simulink subsystem "foc_hall_algorithm"  (R2021b)
settings: Solver=VariableStepAuto  StartTime=0.0  StopTime=10.0  RelTol=1e-3
values from neighbouring files (symbols this model uses):
  PI_params = mcb.internal.SetControllerParameters(pmsm,inverter,PU_System,T_pwm,2*Ts,Ts_speed)    [mcb_pmsm_foc_dual_f28379d_data.m]    (also in mcb_pmsm_foc_dual_f28379d_datascript.m; mcb_pmsm_foc_f280049C_data.m = mcb.internal.SetControllerParameters(pmsm,inverter,PU_System; mcb_pmsm_foc_f28335_data.m = mcb.internal.SetControllerParameters(pmsm,inverter,PU_System; mcb_pmsm_foc_hall_f28035_data.m = mcb.internal.SetControllerParameters(pmsm,inverter,PU_System)
  Ts = 5e-8    (= 5e-08)    [DCDC_Buck_Param.m]    (also in mcb_c2000_open_loop_control_data.m = T_pwm; mcb_c2000_pmsm_offset_data.m = T_pwm; mcb_pmsm_foc_dual_f28379d_data.m = 5e-05; mcb_pmsm_foc_dual_f28379d_datascript.m = 5e-05)
  Ts_speed = 20*Ts    (= 0.001)    [mcb_pmsm_foc_dual_f28379d_data.m]    (also in mcb_pmsm_foc_dual_f28379d_datascript.m; mcb_pmsm_foc_f280049C_data.m = 0.0005; mcb_pmsm_foc_f28335_data.m = 0.0005; mcb_pmsm_foc_hall_f28035_data.m = 0.0005)
libraries: demo_controls x1
settings Model: Creator=The MathWorks, Inc.  LastModifiedBy=The MathWorks, Inc.
settings SolverCC: AlgebraicLoopSolver=TrustRegion
settings DebuggingCC: SFMachineParentedDataDiag=warning

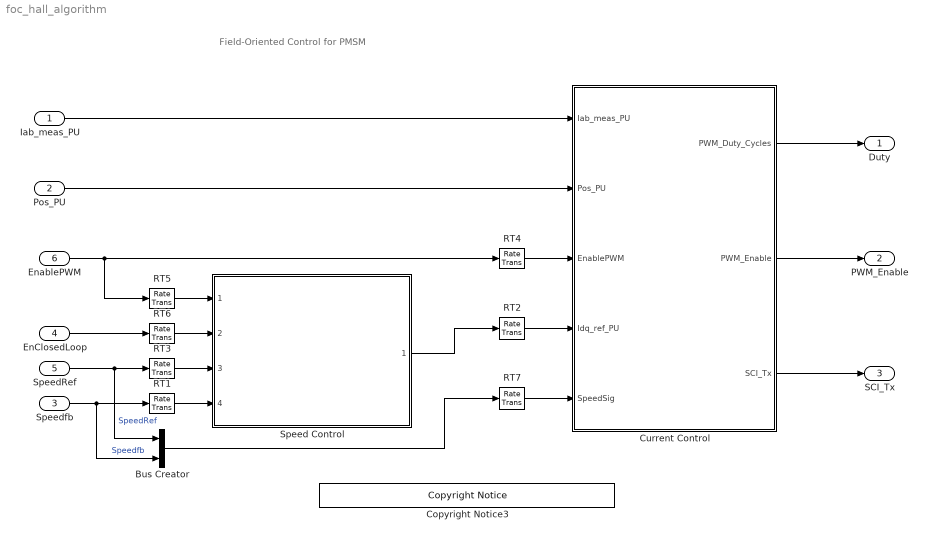
== system foc_hall_algorithm ==
  note: Field-Oriented Control for PMSM
  Iab_meas_PU : Inport
  Pos_PU : Inport  Port=2
  Speedfb : Inport  Port=3
  EnClosedLoop : Inport  Port=4
  SpeedRef : Inport  Port=5
  EnablePWM : Inport  Port=6
  Bus Creator : BusCreator  Inputs=2
  Copyright Notice3 : demo_controls/Copyright Notice  year=2020  prod=tic2000
      settings: SourceProductBaseCode=ME
  Current Control : Subsystem  TreatAsAtomicUnit=on
      settings: RTWSystemCode=Nonreusable function
  RT{1,3,5..6} (4 alike) : RateTransition  Deterministic=off  OutPortSampleTime=Ts_speed
  RT2 : RateTransition  Integrity=off  Deterministic=off  OutPortSampleTime=Ts
  RT4 : RateTransition  Deterministic=off
  RT7 : RateTransition  Integrity=off  Deterministic=off  OutPortSampleTime=Ts
  Speed Control : Subsystem  TreatAsAtomicUnit=on  SystemSampleTime=Ts_speed  ReferencedSubsystem=speed_control  Kp_speed=PI_params.Kp_speed  Ki_speed=PI_params.Ki_speed*Ts_speed
  Duty : Outport  InitialOutput=0  VectorParamsAs1DForOutWhenUnconnected=off
  PWM_Enable : Outport  Port=2  InitialOutput=0  VectorParamsAs1DForOutWhenUnconnected=off
  SCI_Tx : Outport  Port=3  InitialOutput=0  VectorParamsAs1DForOutWhenUnconnected=off
  wires:
  RT6/1 -> Speed Control/2
  Speed Control/1 -> RT2/1
  RT2/1 -> Current Control/4(Idq_ref_PU)
  Current Control/1(PWM_Duty_Cycles) -> Duty/1
  RT1/1 -> Speed Control/4
  RT5/1 -> Speed Control/1
  Current Control/2(PWM_Enable) -> PWM_Enable/1
  Pos_PU/1 -> Current Control/2(Pos_PU)
  RT3/1 -> Speed Control/3
  EnClosedLoop/1 -> RT6/1
  Iab_meas_PU/1 -> Current Control/1(Iab_meas_PU)
  EnablePWM/1 -> RT5/1, RT4/1
  RT4/1 -> Current Control/3(EnablePWM)
  Current Control/3(SCI_Tx) -> SCI_Tx/1
  Bus Creator/1 -> RT7/1
  Speedfb/1 -> Bus Creator/2, RT1/1  "Speedfb"
  SpeedRef/1 -> Bus Creator/1, RT3/1  "SpeedRef"
  RT7/1 -> Current Control/5(SpeedSig)

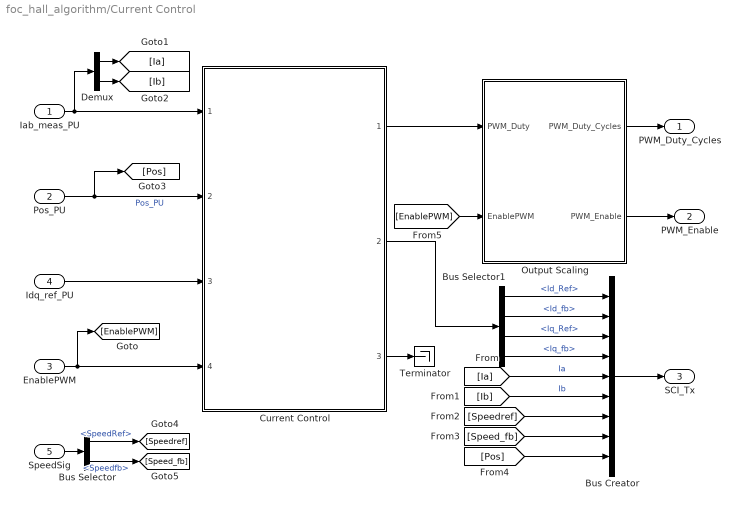
== system foc_hall_algorithm/Current Control ==
  Iab_meas_PU : Inport
  Pos_PU : Inport  Port=2
  EnablePWM : Inport  Port=3
  Idq_ref_PU : Inport  Port=4
  SpeedSig : Inport  Port=5
  Bus Creator : BusCreator  Inputs=9
  Bus Selector : BusSelector  OutputSignals=SpeedRef,Speedfb
  Bus Selector1 : BusSelector  OutputSignals=Id_Ref,Id_fb,Iq_Ref,Iq_fb
  Current Control : Subsystem  ReferencedSubsystem=current_control  Kpd=PI_params.Kp_i  Kid=PI_params.Ki_i*Ts  Kpq=PI_params.Kp_i  Kiq=PI_params.Ki_i*Ts
  Demux : Demux  Outputs=2
  Output Scaling : Subsystem
  Terminator : Terminator
  PWM_Duty_Cycles : Outport
  PWM_Enable : Outport  Port=2
  SCI_Tx : Outport  Port=3
  wires:
  Output Scaling/2(PWM_Enable) -> PWM_Enable/1
  Pos_PU/1 -> [Pos], Current Control/2  "Pos_PU"
  Output Scaling/1(PWM_Duty_Cycles) -> PWM_Duty_Cycles/1
  EnablePWM/1 -> Current Control/4, [EnablePWM]
  Idq_ref_PU/1 -> Current Control/3
  Current Control/1 -> Output Scaling/1(PWM_Duty)
  Iab_meas_PU/1 -> Current Control/1, Demux/1
  [Pos] -> Bus Creator/9
  [Ib] -> Bus Creator/6  "Ib"
  [Speed_fb] -> Bus Creator/8
  Current Control/2 -> Bus Selector1/1
  [Ia] -> Bus Creator/5  "Ia"
  Bus Selector1/4 -> Bus Creator/4  "<Iq_fb>"
  Bus Selector1/3 -> Bus Creator/3  "<Iq_Ref>"
  Bus Selector1/1 -> Bus Creator/1  "<Id_Ref>"
  [Speedref] -> Bus Creator/7
  Bus Selector1/2 -> Bus Creator/2  "<Id_fb>"
  Bus Creator/1 -> SCI_Tx/1
  [EnablePWM] -> Output Scaling/2(EnablePWM)
  Demux/1 -> [Ia]
  Demux/2 -> [Ib]
  SpeedSig/1 -> Bus Selector/1
  Bus Selector/1 -> [Speedref]  "<SpeedRef>"
  Bus Selector/2 -> [Speed_fb]  "<Speedfb>"
  Current Control/3 -> Terminator/1

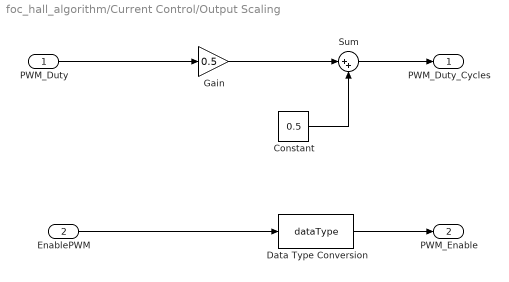
== system foc_hall_algorithm/Current Control/Output Scaling ==
  PWM_Duty : Inport
  EnablePWM : Inport  Port=2
  Constant : Constant  Value=0.5  OutDataTypeStr=dataType
  Data Type Conversion : DataTypeConversion  OutDataTypeStr=dataType
  Gain : Gain  Gain=0.5  OutDataTypeStr=Inherit: Same as input
  Sum : Sum  Inputs=|++
  PWM_Duty_Cycles : Outport
  PWM_Enable : Outport  Port=2
  wires:
  EnablePWM/1 -> Data Type Conversion/1
  Data Type Conversion/1 -> PWM_Enable/1
  PWM_Duty/1 -> Gain/1
  Gain/1 -> Sum/1
  Constant/1 -> Sum/2
  Sum/1 -> PWM_Duty_Cycles/1
